simulink model "sumpModelElegant"  (R2019a)
settings: Solver=VariableStepAuto  StartTime=0.0  StopTime=10.0  RelTol=1e-3
settings Model: Creator=jason.miskin  LastModifiedBy=jason.miskin
settings DataIOCC: ExternalInput=[t, u1,u2,u3,u3]  LoadExternalInput=on

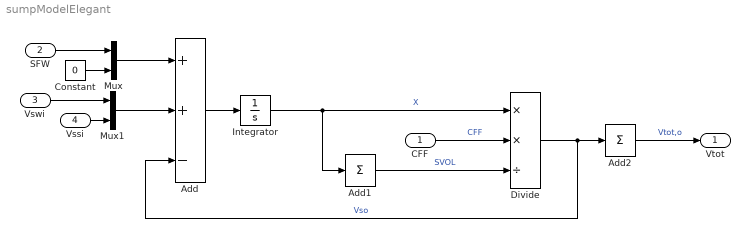
== system sumpModelElegant ==
  CFF : Inport
  SFW : Inport  Port=2
  Vswi : Inport  Port=3
  Vssi : Inport  Port=4
  Add : Sum  Inputs=++-
  Add1 : Sum  Inputs=+
  Add2 : Sum  Inputs=+
  Constant : Constant  Value=0
  Divide : Product  Inputs=**/
  Integrator : Integrator  InitialCondition=[15,15]
  Mux : Mux  Inputs=2
  Mux1 : Mux  Inputs=2
  Vtot : Outport
  wires:
  CFF/1 -> Divide/2  "CFF"
  Add1/1 -> Divide/3  "SVOL"
  Integrator/1 -> Add1/1, Divide/1  "X"
  SFW/1 -> Mux/1
  Vswi/1 -> Mux1/1
  Add/1 -> Integrator/1
  Divide/1 -> Add/3, Add2/1  "Vso"
  Mux/1 -> Add/1
  Constant/1 -> Mux/2
  Vssi/1 -> Mux1/2
  Mux1/1 -> Add/2
  Add2/1 -> Vtot/1  "Vtot,o"
